simulink model "Design1RealTime"  (R2024b)
settings: Solver=FixedStepDiscrete  StartTime=0.0  StopTime=5  FixedStep=0.001  RelTol=1e-3
undefined symbols (not defined in the file): Ao, Bo, Co, Do, K, National_Instruments, Nr, PCI, sens, Ts
libraries: simulink_extras x3, sldrtlib x2
settings Model: SimulationMode=external  ExtModeTrigDuration=1000001  Creator=galeazzolu  LastModifiedBy=galeazzolu
settings DataIOCC: ReturnWorkspaceOutputs=off
settings HardwareCC: ProdBitPerLong=64  ProdHWDeviceType=Intel->x86-64 (Linux 64)
settings RTWCC: Description=Simulink Desktop Real-Time  SystemTargetFile=sldrt.tlc  TemplateMakefile=sldrt.tmf  RTWCompilerOptimization=on
settings CodeAppCC: MaxIdLength=95
settings SimulinkDesktopRealTimeCC: TargetLibSuffix=_sldrt.a  TargetPreCompLibLocation=C:\Program Files\MATLAB\R2024b\toolbox\sldrt\lib\win64  ParMdlRefBuildCompliant=on

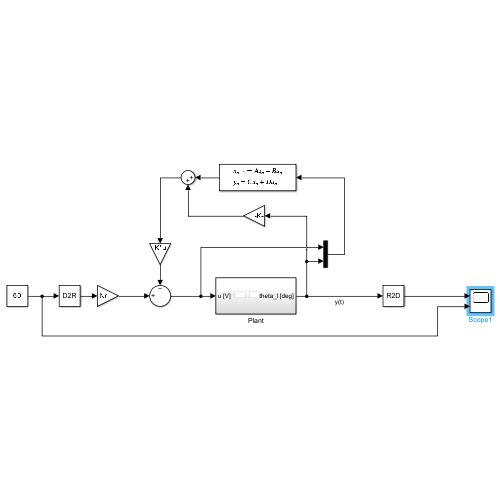
[thumbnail: Simulink's stored preview of the top-level diagram]
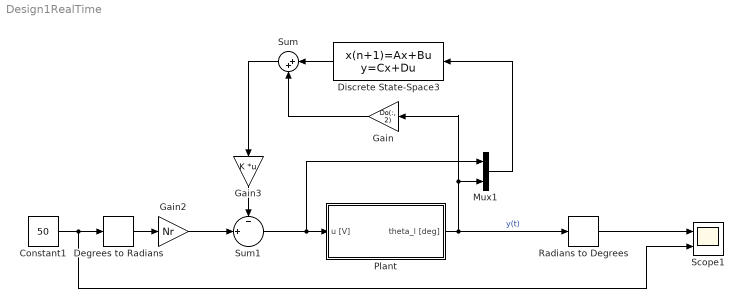
== system Design1RealTime ==
  Constant1 : Constant  Value=50
  Degrees to Radians : simulink_extras/Transformations/Degrees to Radians
  Discrete State-Space3 : DiscreteStateSpace  A=Ao  B=Bo  C=Co  D=zeros(2)  SampleTime=Ts
  Gain : Gain  Gain=Do(:, 2)
  Gain2 : Gain  Gain=Nr
  Gain3 : Gain  Gain=K  Multiplication=Matrix(K*u)
  Mux1 : Mux  Inputs=2
  Plant : Subsystem
  Radians to Degrees : simulink_extras/Transformations/Radians to Degrees
  Scope1 : Scope  NumInputPorts=2
  Sum : Sum  Inputs=|++
  Sum1 : Sum  Inputs=-|+||
  wires:
  Gain2/1 -> Sum1/2
  Discrete State-Space3/1 -> Sum/1
  Gain3/1 -> Sum1/1
  Sum1/1 -> Plant/1(u [V]), Mux1/1
  Constant1/1 -> Scope1/2, Degrees to Radians/1
  Mux1/1 -> Discrete State-Space3/1
  Radians to Degrees/1 -> Scope1/1
  Degrees to Radians/1 -> Gain2/1
  Plant/1(theta_l [deg]) -> Radians to Degrees/1, Mux1/2, Gain/1  "y(t)"
  Sum/1 -> Gain3/1
  Gain/1 -> Sum/2

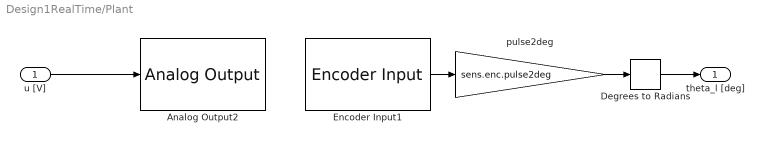
== system Design1RealTime/Plant ==
  u [V] : Inport
  Analog Output2 : sldrtlib/Analog Output  SampleTime=Ts  MaxMissedTicks=10  ShowMissedTicks=off  YieldWhenWaiting=off  DrvName=National_Instruments/PCI-6221  DrvAddress=4294967295  DrvOptions=[0 0 0 2 0]  Channels=1  RangeMode=1  VoltRange=1  InitialValue=0  FinalValue=0
      settings: AttributesFormatString=National Instruments\nPCI-6221 [auto]
  Degrees to Radians : simulink_extras/Transformations/Degrees to Radians
  Encoder Input1 : sldrtlib/Encoder Input  SampleTime=Ts  MaxMissedTicks=10  ShowMissedTicks=off  YieldWhenWaiting=off  DrvName=National_Instruments/PCI-6221  DrvAddress=4294967295  DrvOptions=[0 0 0 2 0]  Channels=1  QuadMode=3  IndexPulse=1  InputFilter=Inf  DataType=1
      settings: AttributesFormatString=National Instruments\nPCI-6221 [auto]
  pulse2deg : Gain  Gain=sens.enc.pulse2deg
  theta_l [deg] : Outport
  wires:
  u [V]/1 -> Analog Output2/1
  Degrees to Radians/1 -> theta_l [deg]/1
  pulse2deg/1 -> Degrees to Radians/1
  Encoder Input1/1 -> pulse2deg/1
